simulink model "Xcvr_SSB_AM_2p5"  (Simulink 8.0)
settings: Solver=VariableStepDiscrete  SolverMode=SingleTasking  StartTime=0.0  StopTime=10  RelTol=1e-3
PreLoadFcn:
  | Fs=80e6;
  | 
  | phee=da_rom();
  | [phee_1,phee_2]=da_i2_rom();
  | 
  | Dcic=64;       % CIC decimation
  | Dfac=128;    % following DA filter decimation
  | N = 6;           %       (2^(N+1))=Dfac
  | Daudio=Dcic*Dfac;
  | Faudio=Fs/Daudio;
  | 
  | load info_filt_ssb_4
  | load Serial_Intfc_Stream_5
  | 
  | % AGC related
  | x=0.5:1/256:(1-1/256);
  | addr=(x-0.5)*256;
  | y=1./x;
values from neighbouring files (symbols this model uses):
  Serial_Interface = [0 0 0 0 0 0 0 0 0 0 0 0 ... (11390 elements, 2x5695)]    [Serial_Intfc_Stream_5.mat]
undefined symbols (not defined in the file or in its folder): get, sided, Two, xlipgetpartsetting
undefined symbols (not defined in the file): ssb_coef
libraries: xbsIndex_r4 x1305, dspsrcs4 x5, simulink x2, dspsigops x2, dspsnks4 x1
(part 3 of 11)

== system Xcvr_SSB_AM_2p5/Audio_and_Mode_Control/T_R_Delay ==
  note: ^ Inserted serial delay here
      | to delay Tx (to help preserve
      | length of iniial CW character, which
      | normally is clipped by about 13 ms).
  Tx_Rx_bit : Inport
  Delay : Inport  Port=2
  Constant1 : xbsIndex_r4/Constant  const=40  gui_display_data_type=Fixed-point  arith_type=Unsigned  n_bits=6  bin_pt=0  preci_type=Single  exp_width=8  frac_width=24  explicit_period=off  period=1  equ=P=C  opselect=C  inp2=PCIN>>17  opr=+  inp1=P  carry=CIN  dbl_ovrd=off  block_type=constant
      settings: block_version=12.1
  Constant2 : xbsIndex_r4/Constant  const=0  gui_display_data_type=Fixed-point  arith_type=Unsigned  n_bits=13  bin_pt=0  preci_type=Single  exp_width=8  frac_width=24  explicit_period=off  period=1  equ=P=C  opselect=C  inp2=PCIN>>17  opr=+  inp1=P  carry=CIN  dbl_ovrd=off  block_type=constant
      settings: block_version=12.1
  Counter : xbsIndex_r4/Counter  cnt_type=Free Running  cnt_to=0  operation=Down  start_count=0  cnt_by_val=1  arith_type=Unsigned  n_bits=12  bin_pt=0  load_pin=on  rst=off  en=on  explicit_period=off  period=1/Faudio  dbl_ovrd=off  use_behavioral_HDL=off  implementation=Fabric  block_type=counter
      settings: block_version=12.1
  Counter1 : xbsIndex_r4/Counter  cnt_type=Free Running  cnt_to=47  operation=Up  start_count=0  cnt_by_val=1  arith_type=Unsigned  n_bits=6  bin_pt=0  load_pin=off  rst=on  en=on  explicit_period=off  period=1  dbl_ovrd=off  use_behavioral_HDL=off  implementation=Fabric  block_type=counter
      settings: block_version=12.1
  Delay1 : xbsIndex_r4/Delay  rst=off  infoeditControl=Selection of Reset will increase slice count due to use of real FFs and instead of SRLs  en=off  latency=160  dbl_ovrd=off  reg_retiming=off  block_type=delay
      settings: block_version=9.2.00
  Delay2 : xbsIndex_r4/Delay  rst=off  infoeditControl=Selection of Reset will increase slice count due to use of real FFs and instead of SRLs  en=off  latency=1  dbl_ovrd=off  reg_retiming=off  block_type=delay
      settings: block_version=9.2.00
  Delay5 : xbsIndex_r4/Delay  rst=off  infoeditControl=Selection of Reset will increase slice count due to use of real FFs and instead of SRLs  en=off  latency=1  dbl_ovrd=off  reg_retiming=off  block_type=delay
      settings: block_version=9.2.00
  Inverter{1..4} (4 alike) : xbsIndex_r4/Inverter  en=off  latency=0  dbl_ovrd=off  block_type=inv
      settings: block_version=9.2.00
  Logical1 : xbsIndex_r4/Logical  logical_function=AND  inputs=2  en=off  latency=0  precision=Full  arith_type=Unsigned  n_bits=16  bin_pt=0  align_bp=on  dbl_ovrd=off  block_type=logical
      settings: block_version=12.1
  Logical2 : xbsIndex_r4/Logical  logical_function=AND  inputs=2  en=off  latency=0  precision=Full  arith_type=Unsigned  n_bits=16  bin_pt=0  align_bp=on  dbl_ovrd=off  block_type=logical
      settings: block_version=12.1
  Logical3 : xbsIndex_r4/Logical  logical_function=OR  inputs=2  en=off  latency=0  precision=Full  arith_type=Unsigned  n_bits=16  bin_pt=0  align_bp=on  dbl_ovrd=off  block_type=logical
      settings: block_version=12.1
  Logical4 : xbsIndex_r4/Logical  logical_function=OR  inputs=3  en=off  latency=0  precision=Full  arith_type=Unsigned  n_bits=16  bin_pt=0  align_bp=on  dbl_ovrd=off  block_type=logical
      settings: block_version=12.1
  Relational : xbsIndex_r4/Relational  mode=a=b  en=off  latency=0  dbl_ovrd=off  block_type=relational
      settings: block_version=9.2.00
  Relational1 : xbsIndex_r4/Relational  mode=a=b  en=off  latency=0  dbl_ovrd=off  block_type=relational
      settings: block_version=9.2.00
  Tx_Rx_D40 : Outport
  Tx_RX : Outport  Port=2
  Tx_RX_Delayed : Outport  Port=3
  wires:
  Tx_Rx_bit/1 -> Delay2/1, Inverter2/1, Logical4/1
  Delay2/1 -> Logical2/2, Logical4/2, Delay1/1
  Constant2/1 -> Relational/2
  Counter/1 -> Relational/1
  Relational/1 -> Inverter1/1
  Inverter1/1 -> Logical3/2, Logical4/3
  Logical3/1 -> Counter/3
  Delay/1 -> Counter/2
  Inverter2/1 -> Logical2/1
  Logical2/1 -> Counter/1, Logical3/1
  Logical4/1 -> Delay5/1
  Delay5/1 -> Tx_RX_Delayed/1, Logical1/1, Inverter3/1
  Counter1/1 -> Relational1/1
  Relational1/1 -> Logical1/2, Inverter4/1
  Inverter3/1 -> Counter1/1
  Constant1/1 -> Relational1/2
  Inverter4/1 -> Counter1/2
  Logical1/1 -> Tx_Rx_D40/1
  Delay1/1 -> Tx_RX/1

== system Xcvr_SSB_AM_2p5/RX Filters D=8192/CIC D64 ==
  note: Select Bits to feed subsequent filters
      | X1  46,44
      | X2  46,43
      | X4 46,42
      | X8 46,41
  I_in : Inport
  Q_in : Inport  Port=2
  CIC Filter : Subsystem  mask(CIC Filter){input_bitwidth=16, input_binpt=15, filter_type=Decimator, rate_change=64, stages=5, m=1, pipeline=on}
      mask prompts: input_bitwidth "Input Bit Width"; input_binpt "Input Binary Point"; filter_type "Filter Type"; rate_change "Sample Rate Change"; stages "Number of Stages"; m "Differential Delay"; pipeline "Pipeline Differentiators"
      mask help: Cascaded Integrated Comb (CIC) Filter
      mask init:
      | % CIC Single Channel v1.0
      | % Set Block Logo
      | sav_gcb=gcb;
      | [bg,fg] = xlcmap('XBlock',0);
      | iPos = get_param(sav_gcb,'Position');
      | iWidth=iPos(3)-iPos(1); iHeight=iPos(4)-iPos(2);
      | iCx=iWidth/2;
      | iCy=iHeight/2;
      | [logoX, logoY] = xlogo(iPos);
      | 
      | % Determine previous filter type and number of stages
      | prev_stages_list = find_system(sav_gcb, 'lookUnderMasks', 'all', 'FollowLinks', 'on', 'Regexp', 'on', 'Name', '^Integrator*'); %this is a cell array
      | prev_stages = length(prev_stages_list);
      | 
      | prev_filter_list = find_system(sav_gcb, 'lookUnderMasks', 'all', 'FollowLinks', 'on', 'Regexp', 'on', 'Name', '^Up Sample*'); %this is a cell array
      | if (isempty(prev_filter_list))
      |     prev_filter_list = find_system(sav_gcb, 'lookUnderMasks', 'all', 'FollowLinks', 'on', 'Regexp', 'on', 'Name', '^Down Sample*'); %this is a cell array
      |     if (isempty(prev_filter_list))
      |         errordlg('Previous Filter Type could not be determined')
      |     else
      |         prev_filter_type = 2;
      |     end
      | else
      |     prev_filter_type = 1;
      | end
      |   
      |   
      | % Print label on the block
      | if(filter_type == 2)
      |    cic_str = sprintf('%d-Stage\n CIC\n%d:1 Decimator',stages, rate_change);
      | else
      |    cic_str = sprintf('%d-Stage\n CIC\n1:%d Interpolator',stages, rate_change);	
      | end
      | 
      | % Make sure the entered values for stages and channels are positive integers
      | nstages = round(sum(abs(stages)));
      | 
      | % issue an error if the number of stages entered is zero
      | if (nstages == 0)
      | 	nstages = prev_stages;
      | 	errordlg('Number of Stages must be more than zero')
      | end
      | 
      | if (nstages == prev_stages) & (filter_type == prev_filter_type)
      |     return
      | end
      | 
      | if(filter_type == 2) % Decimator
      |    if (prev_filter_type == 1) % was interpolator so turn to decimator
      |        for i= 2:prev_stages,
      | 	      delete_line(sav_gcb, ['Integrator' int2str(i-1) '/' int2str(1)], ['Integrator' int2str(i) '/' int2str(1)]);
      | 	      delete_line(sav_gcb, ['Differentiator' int2str(i-1) '/' int2str(1)], ['Differentiator' int2str(i) '/' int2str(1)]);
      |        end
      | 
      |        % disconnect the last blocks in the two sections
      |        delete_line(sav_gcb, ['Differentiator' int2str(prev_stages) '/' int2str(1)], ['Up Sample/1']);
      |        delete_line(sav_gcb, ['Integrator' int2str(prev_stages) '/' int2str(1)], 'Out1/1');
      | 	
      | 	   % delete the line from the Up sampler to the Integrator
      | 	   delete_line(sav_gcb, 'Up Sample/1', 'Integrator1/1'); 
      | 	   delete_line(sav_gcb, 'In1/1', 'Differentiator1/1'); 
      | 	   
      | 	   % Delete the Up Sampler and then replace with an Down Sampler
      | 	   pup = get_param([sav_gcb '/Up Sample'], 'position');
      | 	   delete_block([sav_gcb '/Up Sample']);
      | 	   load_system('xbsIndex_r4');
      | 	   add_block('xbsIndex_r4/Down Sample', [sav_gcb '/Down Sample'], 'sample_ratio', 'rate_change','sample_phase', 'First Value of Frame', 'position', [pup(1), pup(2), pup(3),pup(4)]);
      | 	   
      | 	   % Switch the Integrators and Decimators around
      | 	   for i=1:prev_stages,
      | 		   tempi = get_param([sav_gcb '/Integrator' int2str(i)], 'position');
      | 	       tempd = get_param([sav_gcb '/Differentiator' int2str(i)], 'position');
      | 		   set_param([sav_gcb '/Differentiator' int2str(i)], 'position', [tempi(1), tempi(2), tempi(3), tempi(4)], 'output_bitwidth', 'ceil(stages*log2(rate_change*m) + input_bitwidth)');
      | 		   set_param([sav_gcb '/Integrator' int2str(i)], 'position', [tempd(1), tempd(2), tempd(3), tempd(4)]);
      | 	   end
      | 	   	   	
      | 	   % add back in the lines
      |        add_line(sav_gcb, 'In1/1', 'Integrator1/1', 'autorouting', 'on');
      | 	   add_line(sav_gcb, ['Integrator' int2str(prev_stages) '/1'], 'Down Sample/1', 'autorouting', 'on');
      | 	   add_line(sav_gcb, 'Down Sample/1', 'Differentiator1/1', 'autorouting', 'on');
      | 	   add_line(sav_gcb, ['Differentiator' int2str(prev_stages) '/1'], 'Out1/1', 'autorouting', 'on');
      | 	   for i= 2:prev_stages,
      |           add_line(sav_gcb, ['Integrator' int2str(i-1) '/1'], ['Integrator' int2str(i) '/' int2str(1)], 'autorouting', 'on');
      |           add_line(sav_gcb, ['Differentiator' int2str(i-1) '/1'], ['Differentiator' int2str(i) '/' int2str(1)], 'autorouting', 'on');
      | 	   end
      | 		
      |        %Set the Output bit widths of Differentiator and Integrator stages
      |        set_param([sav_gcb '/Differentiator1'], 'output_bitwidth', 'ceil(stages*log2(rate_change*m) + input_bitwidth)');
      | 	   	   %Set the Output bit width of Integrator stages
      | 	   %Calculate the Interpolator Integrator Output Bit Growth
      |        for i= 1:prev_stages,
      | 			 j = nstages+i;
      | 	         set_param([sav_gcb '/Integrator' int2str(i)], 'output_bitwidth', 'ceil(stages*log2(rate_change*m) + input_bitwidth)');
      |              set_param([sav_gcb '/Differentiator' int2str(i)], 'output_bitwidth', 'ceil(stages*log2(rate_change*m) + input_bitwidth)');
      | 	   end
      | 	   
      |    end
      |    
      |    if (nstages ~= prev_stages)
      |     
      |        % disconnect all the wires from all the blocks
      |        for i= 2:prev_stages,
      | 	      delete_line(sav_gcb, ['Integrator' int2str(i-1) '/' int2str(1)], ['Integrator' int2str(i) '/' int2str(1)]);
      | 	      delete_line(sav_gcb, ['Differentiator' int2str(i-1) '/' int2str(1)], ['Differentiator' int2str(i) '/' int2str(1)]);
      |        end
      | 
      |        % disconnect the last blocks in the two sections
      |        delete_line(sav_gcb, ['Integrator' int2str(prev_stages) '/' int2str(1)], ['Down Sample/1']);
      |        delete_line(sav_gcb, ['Differentiator' int2str(prev_stages) '/' int2str(1)], 'Out1/1');
      | 	
      | 	   % delete the line from the down sampler to the differentiator
      | 	   delete_line(sav_gcb, 'Down Sample/1', 'Differentiator1/1');
      | 	
      | 	   % Remove all the blocks except the first one (as we always will have one)
      |        for i=2:prev_stages,
      | 		  delete_block([sav_gcb '/Differentiator' int2str(i)]);
      | 	      delete_block([sav_gcb '/Integrator' int2str(i)]);
      |        end
      | 	   
      | 	   %Set the Output bit width of Differentiator stages
      |        set_param([sav_gcb '/Differentiator1'], 'output_bitwidth', 'ceil(stages*log2(rate_change*m) + input_bitwidth)');
      | 	   
      | 	   % collect data on the position of existing blocks
      | 	   pi = get_param([sav_gcb '/Integrator1'], 'position');
      | 	   pd = get_param([sav_gcb '/Differentiator1'], 'position');
      | 	   set_param([sav_gcb '/Differentiator1'], 'position', [pi(1)+(nstages+1)*80, pd(2), pi(3)+(nstages+1)*80, pd(4)]);
      | 	   pd = get_param([sav_gcb '/Differentiator1'], 'position');
      | 	
      | 	   % move the current blocks to accomadate for new blocks to be added 
      | 	   pds = get_param([sav_gcb '/Down Sample'], 'position');
      | 	   set_param([sav_gcb '/Down Sample'], 'position', [pi(1)+(nstages)*80, pds(2), pi(3)+(nstages)*80, pds(4)]);
      | 	   
      | 	   po = get_param([sav_gcb '/Out1'], 'position');
      | 	   set_param([sav_gcb '/Out1'], 'position', [pd(1)+(nstages+1)*80, po(2), pd(1)+(po(3)-po(1))+(nstages+1)*80, po(4)]);	
      | 	
      | 	   % add back in the line between the Down Sampler and the 1st Differentiator
      |        add_line(sav_gcb, 'Down Sample/1', ['Differentiator1/' int2str(1)], 'autorouting', 'on');
      | 
      | 	   % Only add blocks if more than one stage is required
      | 	   if (nstages ~= 1)
      | 		
      | 	       % Add in a copy of the first block to make up the required number of stages
      |            for i=2:nstages,
      |                add_block([sav_gcb '/Integrator1'], [sav_gcb '/Integrator' int2str(i)], 'position', [pi(1)+(i-1)*80, pi(2), pi(3)+(i-1)*80, pi(4)]);
      | 		       add_block([sav_gcb '/Differentiator1'], [sav_gcb '/Differentiator' int2str(i)], 'position', [pd(1)+(i-1)*80, pd(2), pd(3)+(i-1)*80, pd(4)]);
      | 	       end
      | 		
      | 	       % Connect up the wires to each block use autorouting
      |            for i= 2:nstages,
      |  		       add_line(sav_gcb, ['Integrator' int2str(i-1) '/' int2str(1)], ['Integrator' int2str(i) '/' int2str(1)], 'autorouting', 'on');
      | 	           add_line(sav_gcb, ['Differentiator' int2str(i-1) '/' int2str(1)], ['Differentiator' int2str(i) '/' int2str(1)], 'autorouting', 'on');
      |            end
      | 	    end
      | 	       % Connect the last blocks in the two sections
      |            add_line(sav_gcb, ['Integrator' int2str(nstages) '/' int2str(1)], ['Down Sample/1'], 'autorouting', 'on');
      |            add_line(sav_gcb, ['Differentiator' int2str(nstages) '/' int2str(1)], ['Out1/1'], 'autorouting', 'on');
      |    end
      | 
      | else % Interpolator
      |    
      | 	
      | 	if (prev_filter_type == 2) % was decimator so turn to interpolator
      | 	
      | 	  % disconnect all the wires from all the blocks
      |        for i= 2:prev_stages,
      | 	      delete_line(sav_gcb, ['Integrator' int2str(i-1) '/' int2str(1)], ['Integrator' int2str(i) '/' int2str(1)]);
      | 	      delete_line(sav_gcb, ['Differentiator' int2str(i-1) '/' int2str(1)], ['Differentiator' int2str(i) '/' int2str(1)]);
      |        end
      | 
      |        % disconnect the last blocks in the two sections
      |        delete_line(sav_gcb, ['Integrator' int2str(prev_stages) '/' int2str(1)], ['Down Sample/1']);
      |        delete_line(sav_gcb, ['Differentiator' int2str(prev_stages) '/' int2str(1)], 'Out1/1');
      | 	
      | 	   % delete the line from the down sampler to the Differentiator
      | 	   delete_line(sav_gcb, 'Down Sample/1', 'Differentiator1/1'); 
      | 	   delete_line(sav_gcb, 'In1/1', 'Integrator1/1'); 
      | 	   
      | 	   % Delete the Down Sampler and then replace with a Up Sampler
      | 	   pdwn = get_param([sav_gcb '/Down Sample'], 'position');
      | 	   delete_block([sav_gcb '/Down Sample']);
      | 	   load_system('xbsIndex_r4');
      | 	   add_block('xbsIndex_r4/Up Sample', [sav_gcb '/Up Sample'], 'sample_ratio', 'rate_change', 'position', [pdwn(1), pdwn(2), pdwn(3), pdwn(4)]);
      | 	   
      | 	   % Switch the Integrators and Decimators around
      | 	   for i=1:prev_stages,
      | 		   tempi = get_param([sav_gcb '/Integrator' int2str(i)], 'position');
      | 	       tempd = get_param([sav_gcb '/Differentiator' int2str(i)], 'position');
      | 		   set_param([sav_gcb '/Differentiator' int2str(i)], 'position', [tempi(1), tempi(2), tempi(3), tempi(4)], 'output_bitwidth', [int2str(i) '+ input_bitwidth']);
      | 		   set_param([sav_gcb '/Integrator' int2str(i)], 'position', [tempd(1), tempd(2), tempd(3), tempd(4)]);
      | 	   end
      | 	   	   	
      | 	   % add back in the lines
      |        add_line(sav_gcb, 'In1/1', 'Differentiator1/1', 'autorouting', 'on');
      | 	   add_line(sav_gcb, ['Differentiator' int2str(prev_stages) '/1'], 'Up Sample/1', 'autorouting', 'on');
      | 	   add_line(sav_gcb, 'Up Sample/1', 'Integrator1/1', 'autorouting', 'on');
      | 	   add_line(sav_gcb, ['Integrator' int2str(prev_stages) '/1'], 'Out1/1', 'autorouting', 'on');
      | 	   for i= 2:prev_stages,
      |           add_line(sav_gcb, ['Integrator' int2str(i-1) '/1'], ['Integrator' int2str(i) '/1'], 'autorouting', 'on');
      |           add_line(sav_gcb, ['Differentiator' int2str(i-1) '/1'], ['Differentiator' int2str(i) '/1'], 'autorouting', 'on');
      | 	   end
      | 	   
      | 	   %Set the Output bit width of Integrator stages
      | 	   %Calculate the Interpolator Integrator Output Bit Growth
      |        for i= 1:prev_stages,
      | 			 j = nstages+i;
      | 	         set_param([sav_gcb '/Integrator' int2str(i)], 'output_bitwidth', ['ceil(log2(2^(2*stages-' int2str(j) ')*(rate_change*m)^(' int2str(j) '-stages)) + input_bitwidth)']);
      | 	   end
      | 		
      |    end
      |    
      | 	
      | 	if (nstages ~= prev_stages)
      |     
      |        % disconnect all the wires from all the blocks
      |        for i= 2:prev_stages,
      | 	      delete_line(sav_gcb, ['Integrator' int2str(i-1) '/' int2str(1)], ['Integrator' int2str(i) '/' int2str(1)]);
      | 	      delete_line(sav_gcb, ['Differentiator' int2str(i-1) '/' int2str(1)], ['Differentiator' int2str(i) '/' int2str(1)]);
      |        end
      | 
      |        % disconnect the last blocks in the two sections
      |        delete_line(sav_gcb, ['Differentiator' int2str(prev_stages) '/' int2str(1)], ['Up Sample/1']);
      |        delete_line(sav_gcb, ['Integrator' int2str(prev_stages) '/' int2str(1)], 'Out1/1');
      |        
      | 	
      | 	   % delete the line from the Up sampler to the Integrator1 for movement later
      | 	   delete_line(sav_gcb, 'Up Sample/1', 'Integrator1/1'); 
      | 	
      | 	   % Remove all the blocks except the first one (as we always will have one)
      |        for i=2:prev_stages,
      | 		  delete_block([sav_gcb '/Differentiator' int2str(i)]);
      | 	      delete_block([sav_gcb '/Integrator' int2str(i)]);
      |        end
      | 	
      | 	   %Set the Output bit width of first Differentiator stage (other are set as copies of this block)
      |        set_param([sav_gcb '/Differentiator1'], 'output_bitwidth', '1 + input_bitwidth');
      | 	   
      | 	   % collect data on the position of existing blocks
      | 	   pi = get_param([sav_gcb '/Integrator1'], 'position');
      | 	   pd = get_param([sav_gcb '/Differentiator1'], 'position');
      | 	   set_param([sav_gcb '/Integrator1'], 'position', [pd(1)+(nstages+1)*80, pi(2), pd(3)+(nstages+1)*80, pi(4)]);
      | 	   pi = get_param([sav_gcb '/Integrator1'], 'position');
      | 	
      | 	   % move the current blocks to accomadate for new blocks to be added 
      | 	   pus = get_param([sav_gcb '/Up Sample'], 'position');
      | 	   set_param([sav_gcb '/Up Sample'], 'position', [pd(1)+(nstages)*80, pus(2), pd(3)+(nstages)*80, pus(4)]);
      | 	
      | 	   po = get_param([sav_gcb '/Out1'], 'position');
      |        set_param([sav_gcb '/Out1'], 'position', [pi(1)+(nstages+1)*80, po(2), pi(1)+(po(3)-po(1))+(nstages+1)*80, po(4)]);	
      |       
      | 	
      | 	   % add back in the line between the Up Sampler and the 1st Integrator1
      | 	   add_line(sav_gcb, 'Up Sample/1', 'Integrator1/1', 'autorouting', 'on');
      | 	   
      | 	   % Only add blocks if more than one stage is required
      | 	   if (nstages ~= 1)
      | 		
      | 	       % Add in a copy of the first block to make up the required number of stages
      |            for i=2:nstages,
      |                add_block([sav_gcb '/Integrator1'], [sav_gcb '/Integrator' int2str(i)], 'position', [pi(1)+(i-1)*80, pi(2), pi(3)+(i-1)*80, pi(4)]);
      | 		       add_block([sav_gcb '/Differentiator1'], [sav_gcb '/Differentiator' int2str(i)], 'position', [pd(1)+(i-1)*80, pd(2), pd(3)+(i-1)*80, pd(4)], 'output_bitwidth', [int2str(i) '+ input_bitwidth']);
      | 	       end
      | 		
      | 	       % Connect up the wires to each block use autorouting
      |            for i= 2:nstages,
      |  		       add_line(sav_gcb, ['Integrator' int2str(i-1) '/' int2str(1)], ['Integrator' int2str(i) '/' int2str(1)], 'autorouting', 'on');
      | 	           add_line(sav_gcb, ['Differentiator' int2str(i-1) '/' int2str(1)], ['Differentiator' int2str(i) '/' int2str(1)], 'autorouting', 'on');
      |            end
      | 	    end
      | 	       % Connect the last blocks in the two sections
      |            add_line(sav_gcb, ['Differentiator' int2str(nstages) '/1'], ['Up Sample/1'], 'autorouting', 'on');
      |            add_line(sav_gcb, ['Integrator' int2str(nstages) '/1'], ['Out1/1'], 'autorouting', 'on');
      | 		   
      | 	     %Set the Output bit width of Integrator stages
      | 	     %Calculate the Interpolator Integrator Output Bit Growth
      |           for i= 1:nstages,
      | 			 j = nstages+i;
      | 	         set_param([sav_gcb '/Integrator' int2str(i)], 'output_bitwidth', ['ceil(log2(2^(2*stages-' int2str(j) ')*(rate_change*m)^(' int2str(j) '-stages)) + input_bitwidth)']);
      | 	      end
      |    end
      | 	  
      | end
      | 
      | 
      | % Set the pipelining to ON or OFF on the differentiators
      | if (pipeline == 0)
      | 	for i= 1:nstages
      | 		set_param([sav_gcb '/Differentiator' int2str(i), '/AddSub'], 'latency', '0')
      | 	end
      | else
      | 	for i= 1:nstages
      | 		set_param([sav_gcb '/Differentiator' int2str(i), '/AddSub'], 'latency' ,'1')
      | 	end
      | end
      settings: CopyFcn=set_param(gcb, 'MaskSelfModifiable', 'on', 'LinkStatus', 'none');
      mask Help: eval('');xlDoc('-book','sysgen','-topic','CIC_Filter');
      mask TypeOptions filter_type: Interpolator | Decimator
      mask TypeOptions m: 1 | 2 | 3 | 4
      mask Display:
      | patch([0 iWidth iWidth 0],[0 0 iHeight iHeight] , bg);
      | patch(logoX,logoY , fg);
      | plot([0 0 iWidth iWidth 0], [0 iHeight iHeight 0 0]);
      | disp(cic_str)
  CIC Filter1 : Subsystem  mask(CIC Filter){input_bitwidth=16, input_binpt=15, filter_type=Decimator, rate_change=64, stages=5, m=1, pipeline=on}
      mask prompts: input_bitwidth "Input Bit Width"; input_binpt "Input Binary Point"; filter_type "Filter Type"; rate_change "Sample Rate Change"; stages "Number of Stages"; m "Differential Delay"; pipeline "Pipeline Differentiators"
      mask help: Cascaded Integrated Comb (CIC) Filter
      mask init: same as Xcvr_SSB_AM_2p5/RX Filters D=8192/CIC D64/CIC Filter
      settings: CopyFcn=set_param(gcb, 'MaskSelfModifiable', 'on', 'LinkStatus', 'none');
      mask Help: eval('');xlDoc('-book','sysgen','-topic','CIC_Filter');
      mask TypeOptions filter_type: Interpolator | Decimator
      mask TypeOptions m: 1 | 2 | 3 | 4
      mask Display:
      | patch([0 iWidth iWidth 0],[0 0 iHeight iHeight] , bg);
      | patch(logoX,logoY , fg);
      | plot([0 0 iWidth iWidth 0], [0 iHeight iHeight 0 0]);
      | disp(cic_str)
  Convert1 : xbsIndex_r4/Convert  gui_display_data_type=Fixed-point  arith_type="Signed  (2's comp)"  n_bits=21  bin_pt=20  float_type=Single  exp_bits=8  fraction_bits=24  quantization="Round  (unbiased: +/- Inf)"  overflow=Saturate  en=off  latency=1  dbl_ovrd=off  pipeline=off  block_type=convert
      settings: block_version=9.2.00
  Convert2 : xbsIndex_r4/Convert  gui_display_data_type=Fixed-point  arith_type="Signed  (2's comp)"  n_bits=21  bin_pt=20  float_type=Single  exp_bits=8  fraction_bits=24  quantization="Round  (unbiased: +/- Inf)"  overflow=Saturate  en=off  latency=1  dbl_ovrd=off  pipeline=off  block_type=convert
      settings: block_version=9.2.00
  OverLoad_Det : Subsystem
  Reinterpret  X1a : xbsIndex_r4/Reinterpret  force_arith_type=on  arith_type="Signed  (2's comp)"  force_bin_pt=on  bin_pt=44  block_type=reinterpret
      settings: infoedit="Changes signal type without altering the binary representation.   You can changed the signal between signed and unsigned, and relocate the binary point.<br><br>Hardware notes: In hardware this block costs nothing.<br><br>Example:  Suppose the input is 6 bits wide, signed, with 2 fractional bits, and the output is forced to unsigned with 0 fractional bits.  Then an input of -2.0 (1110.00 in binary 2's complement) becomes an output of 56 (111000 in binary)."  block_version=9.2.00
  Reinterpret1 : xbsIndex_r4/Reinterpret  force_arith_type=on  arith_type="Signed  (2's comp)"  force_bin_pt=on  bin_pt=44  block_type=reinterpret
      settings: infoedit="Changes signal type without altering the binary representation.   You can changed the signal between signed and unsigned, and relocate the binary point.<br><br>Hardware notes: In hardware this block costs nothing.<br><br>Example:  Suppose the input is 6 bits wide, signed, with 2 fractional bits, and the output is forced to unsigned with 0 fractional bits.  Then an input of -2.0 (1110.00 in binary 2's complement) becomes an output of 56 (111000 in binary)."  block_version=9.2.00
  I_Out : Outport
  Q_Out : Outport  Port=2
  CIC_Ovl : Outport  Port=3
  wires:
  CIC Filter/1(Out1) -> Reinterpret  X1a/1
  Reinterpret  X1a/1 -> Convert2/1
  I_in/1 -> CIC Filter/1(In1)
  Q_in/1 -> CIC Filter1/1(In1)
  Convert2/1 -> I_Out/1, OverLoad_Det/1(In1)  "I_X1"
  CIC Filter1/1(Out1) -> Reinterpret1/1
  Reinterpret1/1 -> Convert1/1
  OverLoad_Det/1(Out1) -> CIC_Ovl/1
  Convert1/1 -> Q_Out/1  "Q_X1"

== system Xcvr_SSB_AM_2p5/RX Filters D=8192/DA_Ovl_Det ==
  In1 : Inport
  Constant : xbsIndex_r4/Constant  const=0  gui_display_data_type=Fixed-point  arith_type=Unsigned  n_bits=8  bin_pt=0  preci_type=Single  exp_width=8  frac_width=24  explicit_period=off  period=1  equ=P=C  opselect=C  inp2=PCIN>>17  opr=+  inp1=P  carry=CIN  dbl_ovrd=off  block_type=constant
      settings: block_version=9.2.00
  Counter : xbsIndex_r4/Counter  cnt_type=Free Running  cnt_to=Inf  operation=Up  start_count=0  cnt_by_val=1  arith_type=Unsigned  n_bits=8  bin_pt=0  load_pin=off  rst=off  en=off  explicit_period=on  period=8192/Fs  dbl_ovrd=off  use_behavioral_HDL=off  implementation=Fabric  use_rpm=off  block_type=counter
      settings: block_version=9.2.00
  Inverter{,1..3} (4 alike) : xbsIndex_r4/Inverter  en=off  latency=0  dbl_ovrd=off  block_type=inv
      settings: block_version=9.2.00
  Logical : xbsIndex_r4/Logical  logical_function=AND  inputs=4  en=off  latency=0  precision=Full  arith_type=Unsigned  n_bits=16  bin_pt=0  align_bp=on  dbl_ovrd=off  block_type=logical
      settings: block_version=9.2.00
  Logical1 : xbsIndex_r4/Logical  logical_function=AND  inputs=4  en=off  latency=0  precision=Full  arith_type=Unsigned  n_bits=16  bin_pt=0  align_bp=on  dbl_ovrd=off  block_type=logical
      settings: block_version=9.2.00
  Logical2 : xbsIndex_r4/Logical  logical_function=OR  inputs=2  en=off  latency=1  precision=Full  arith_type=Unsigned  n_bits=16  bin_pt=0  align_bp=on  dbl_ovrd=off  block_type=logical
      settings: block_version=9.2.00
  Logical3 : xbsIndex_r4/Logical  logical_function=OR  inputs=2  en=off  latency=0  precision=Full  arith_type=Unsigned  n_bits=16  bin_pt=0  align_bp=on  dbl_ovrd=off  block_type=logical
      settings: block_version=9.2.00
  Register : xbsIndex_r4/Register  init=0  rst=on  en=off  dbl_ovrd=off  block_type=register
      settings: block_version=9.2.00
  Relational : xbsIndex_r4/Relational  mode=a=b  en=off  latency=0  dbl_ovrd=off  block_type=relational
      settings: block_version=9.2.00
  Slice : xbsIndex_r4/Slice  nbits=1  boolean_output=on  mode=Upper Bit Location + Width  bit1=0  base1=MSB of Input  bit0=0  base0=LSB of Input  dbl_ovrd=off  block_type=slice
      settings: infoedit="Extracts a given range of bits from each input sample and presents it at the output.  The output type is ordinarily unsigned with binary point at zero, but can be Boolean when the slice is one bit wide.<P><P>Hardware notes: In hardware this block costs nothing."  block_version=9.2.00
  Slice1 : xbsIndex_r4/Slice  nbits=1  boolean_output=on  mode=Upper Bit Location + Width  bit1=-1  base1=MSB of Input  bit0=0  base0=LSB of Input  dbl_ovrd=off  block_type=slice
      settings: infoedit="Extracts a given range of bits from each input sample and presents it at the output.  The output type is ordinarily unsigned with binary point at zero, but can be Boolean when the slice is one bit wide.<P><P>Hardware notes: In hardware this block costs nothing."  block_version=9.2.00
  Slice2 : xbsIndex_r4/Slice  nbits=1  boolean_output=on  mode=Upper Bit Location + Width  bit1=-2  base1=MSB of Input  bit0=0  base0=LSB of Input  dbl_ovrd=off  block_type=slice
      settings: infoedit="Extracts a given range of bits from each input sample and presents it at the output.  The output type is ordinarily unsigned with binary point at zero, but can be Boolean when the slice is one bit wide.<P><P>Hardware notes: In hardware this block costs nothing."  block_version=9.2.00
  Slice3 : xbsIndex_r4/Slice  nbits=1  boolean_output=on  mode=Upper Bit Location + Width  bit1=-3  base1=MSB of Input  bit0=0  base0=LSB of Input  dbl_ovrd=off  block_type=slice
      settings: infoedit="Extracts a given range of bits from each input sample and presents it at the output.  The output type is ordinarily unsigned with binary point at zero, but can be Boolean when the slice is one bit wide.<P><P>Hardware notes: In hardware this block costs nothing."  block_version=9.2.00
  Out1 : Outport
  wires:
  Slice/1 -> Inverter/1, Logical1/1
  In1/1 -> Slice/1, Slice1/1, Slice2/1, Slice3/1
  Inverter/1 -> Logical/1
  Slice1/1 -> Logical/2, Inverter1/1
  Slice2/1 -> Logical/3, Inverter2/1
  Slice3/1 -> Logical/4, Inverter3/1
  Inverter1/1 -> Logical1/2
  Inverter2/1 -> Logical1/3
  Inverter3/1 -> Logical1/4
  Logical1/1 -> Logical2/2
  Logical/1 -> Logical2/1
  Logical2/1 -> Logical3/1
  Logical3/1 -> Register/1
  Register/1 -> Out1/1, Logical3/2
  Relational/1 -> Register/2
  Counter/1 -> Relational/1
  Constant/1 -> Relational/2

== system Xcvr_SSB_AM_2p5/RX Filters D=8192/Decimating Filter DC Optimized in Accumulator Plus Pipelined Stage Control. Improved dynamic  range.  ==
  Real_In : Inport
  Imag_In : Inport  Port=2
  Dfac : Inport  Port=3
  D=2 Bit Serial Filter Core with Piplined RAM Based SR : Subsystem
  Interstage  Interface1 : Subsystem
  Real_Imag_Demux1 : Subsystem
  Reinterpret2 : xbsIndex_r4/Reinterpret  force_arith_type=on  arith_type="Signed  (2's comp)"  force_bin_pt=on  bin_pt=20  block_type=reinterpret
      settings: infoedit="Changes signal type without altering the binary representation.   You can changed the signal between signed and unsigned, and relocate the binary point.<br><br>Hardware notes: In hardware this block costs nothing.<br><br>Example:  Suppose the input is 6 bits wide, signed, with 2 fractional bits, and the output is forced to unsigned with 0 fractional bits.  Then an input of -2.0 (1110.00 in binary 2's complement) becomes an output of 56 (111000 in binary)."  block_version=9.2.00
  Reinterpret3 : xbsIndex_r4/Reinterpret  force_arith_type=on  arith_type="Signed  (2's comp)"  force_bin_pt=on  bin_pt=0  block_type=reinterpret
      settings: infoedit="Changes signal type without altering the binary representation.   You can changed the signal between signed and unsigned, and relocate the binary point.<P><P>Hardware notes: In hardware this block costs nothing.<P><P>Example:  Suppose the input is 6 bits wide, signed, with 2 fractional bits, and the output is forced to unsigned with 0 fractional bits.  Then an input of -2.0 (1110.00 in binary 2's complement) becomes an output of 56 (111000 in binary)."  block_version=9.2.00
  Reinterpret4 : xbsIndex_r4/Reinterpret  force_arith_type=on  arith_type="Signed  (2's comp)"  force_bin_pt=on  bin_pt=20  block_type=reinterpret
      settings: infoedit="Changes signal type without altering the binary representation.   You can changed the signal between signed and unsigned, and relocate the binary point.<br><br>Hardware notes: In hardware this block costs nothing.<br><br>Example:  Suppose the input is 6 bits wide, signed, with 2 fractional bits, and the output is forced to unsigned with 0 fractional bits.  Then an input of -2.0 (1110.00 in binary 2's complement) becomes an output of 56 (111000 in binary)."  block_version=9.2.00
  Reinterpret5 : xbsIndex_r4/Reinterpret  force_arith_type=on  arith_type="Signed  (2's comp)"  force_bin_pt=on  bin_pt=0  block_type=reinterpret
      settings: infoedit="Changes signal type without altering the binary representation.   You can changed the signal between signed and unsigned, and relocate the binary point.<P><P>Hardware notes: In hardware this block costs nothing.<P><P>Example:  Suppose the input is 6 bits wide, signed, with 2 fractional bits, and the output is forced to unsigned with 0 fractional bits.  Then an input of -2.0 (1110.00 in binary 2's complement) becomes an output of 56 (111000 in binary)."  block_version=9.2.00
  Relational : xbsIndex_r4/Relational  mode=a=b  en=off  latency=0  dbl_ovrd=off  block_type=relational
      settings: block_version=9.2.00
  Stage Control with Pipe : Subsystem
  Terminator1 : Terminator
  Real_Out : Outport
  Imag_Out : Outport  Port=2
  wires:
  Reinterpret4/1 -> Imag_Out/1
  Stage Control with Pipe/2(SR_addr) -> D=2 Bit Serial Filter Core with Piplined RAM Based SR/3(SR_addr)
  Stage Control with Pipe/3(Real_Imag) -> Interstage  Interface1/7(Real_Imag), Real_Imag_Demux1/3(Real_Imag)
  Stage Control with Pipe/1(AB_Addr) -> Interstage  Interface1/5(AB_Addr)
  Stage Control with Pipe/5(Write_OK) -> Interstage  Interface1/8(Write_OK)
  D=2 Bit Serial Filter Core with Piplined RAM Based SR/1(Yn) -> Real_Imag_Demux1/1(Yn), Interstage  Interface1/1(Previous Stage)
  D=2 Bit Serial Filter Core with Piplined RAM Based SR/2(Valid) -> Interstage  Interface1/2(Write), Real_Imag_Demux1/2(Valid_In)
  Stage Control with Pipe/6(Start) -> D=2 Bit Serial Filter Core with Piplined RAM Based SR/4(Start)
  Stage Control with Pipe/7(Stage) -> Relational/1
  Relational/1 -> Real_Imag_Demux1/4(Stage_Sel)
  Real_In/1 -> Reinterpret3/1
  Real_Imag_Demux1/1(Real) -> Reinterpret2/1  "Real"
  Real_Imag_Demux1/2(Imag) -> Reinterpret4/1
  Real_Imag_Demux1/3(Valid) -> Terminator1/1  "Valid"
  Reinterpret3/1 -> Interstage  Interface1/3(Real_In)
  Reinterpret5/1 -> Interstage  Interface1/4(Imag_In)
  Imag_In/1 -> Reinterpret5/1
  Stage Control with Pipe/4(Stage>0) -> Interstage  Interface1/6(Stage>0)
  Interstage  Interface1/1(Xn) -> D=2 Bit Serial Filter Core with Piplined RAM Based SR/1(Xn)
  Interstage  Interface1/2(Xn-1) -> D=2 Bit Serial Filter Core with Piplined RAM Based SR/2(Xn-1)
  Reinterpret2/1 -> Real_Out/1
  Dfac/1 -> Relational/2

== system Xcvr_SSB_AM_2p5/RX Filters D=8192/Fs_probe ==
  In1 : Inport
  Probe : Probe  ProbeWidth=off  ProbeComplexSignal=off
  Product : Product  Inputs=/  RndMeth=Zero
  Selector : Selector  InputPortWidth=2  IndexOptions=Index vector (dialog)  Indices=1  OutputSizes=1
  Out1 : Outport
  wires:
  Selector/1 -> Product/1
  Probe/1 -> Selector/1
  In1/1 -> Probe/1
  Product/1 -> Out1/1

== system Xcvr_SSB_AM_2p5/SSB / AM Mod_Demod WCS/128 Tap FIR with  Writable Coefficient Store ==
  note: [15 14 13 12 .... 3 2 1 0] [5 4 3 2 1 0] [Bank_Sel] [Reset], [WE] X
  note: 16 Data 6 Address Bank Select Reset Write Enable X
  note: 25 24 23 22 ....13 12 11 10 9 8 7 6 5 4 3 2 1 0
  note: Added delay 7/31/2016
  note: To load WCS:
      | 1) Set Reset Bit then in a loop...
      | 2) With both Reset and WE set,
      | load 6 address and 16 Data bits. 64X for entire RAM.
      | 3) Lower both Reset and WE.
      | Yes one bit could do the job.
  I_In : Inport
  Q_In : Inport  Port=2
  Data_26 : Inport  Port=3
  WR_COEF_RAM : Inport  Port=4
  Tx_Rx_Delayed : Inport  Port=5
  2 channel (IQ)  SHARED MPY MAC with Writable Coefficient Store : Subsystem  mask(2n-tap Linear Phase MAC FIR Filter){coef=ssb_coef, coef_n_bits=16, coef_bin_pt=16, smpl_n_bits=18, smpl_bin_pt=17, smpl_period=Daudio/Fs}
      mask prompts: coef "Coefficients_1"; coef_n_bits "Number of Bits per Coefficient"; coef_bin_pt "Binary Point for Coefficient"; smpl_n_bits "Number of Bits per Input Sample"; smpl_bin_pt "Binary Point for Input Samples"; smpl_period "Input Sample Period"
      mask help:
      | Linear phase MAC-based FIR filter with 2*n coefficients.
      | Design exploits even coefficient symmetry.
      mask init:
      | dstr = sprintf('%d tap',length(coef));
  Address_Slice : xbsIndex_r4/Slice  nbits=6  boolean_output=off  mode=Lower Bit Location + Width  bit1=-17  base1=LSB of Input  bit0=4  base0=LSB of Input  dbl_ovrd=off  block_type=slice
      settings: block_version=12.1
  Bank_Sel : xbsIndex_r4/Slice  nbits=1  boolean_output=on  mode=Lower Bit Location + Width  bit1=-17  base1=LSB of Input  bit0=3  base0=LSB of Input  dbl_ovrd=off  block_type=slice
      settings: block_version=12.1
  Data_Slice : xbsIndex_r4/Slice  nbits=16  boolean_output=off  mode=Lower Bit Location + Width  bit1=-17  base1=LSB of Input  bit0=10  base0=LSB of Input  dbl_ovrd=off  block_type=slice
      settings: block_version=12.1
  Down Sample : xbsIndex_r4/Down Sample  sample_ratio=1024/4  sample_phase="Last Value of Frame  (most efficient)"  en=off  latency=1  dbl_ovrd=off  block_type=dsamp
      settings: block_version=9.2.00
  Down Sample1 : xbsIndex_r4/Down Sample  sample_ratio=256  sample_phase=First Value of Frame  en=off  latency=0  dbl_ovrd=off  block_type=dsamp
      settings: block_version=9.2.00
  Information_Filter_Transient_Suppressor : Subsystem
  Logical : xbsIndex_r4/Logical  logical_function=OR  inputs=2  en=off  latency=0  precision=Full  arith_type=Unsigned  n_bits=16  bin_pt=0  align_bp=on  dbl_ovrd=off  block_type=logical
      settings: block_version=9.2.00
  Logical1 : xbsIndex_r4/Logical  logical_function=AND  inputs=2  en=off  latency=1  precision=Full  arith_type=Unsigned  n_bits=16  bin_pt=0  align_bp=on  dbl_ovrd=off  block_type=logical
      settings: block_version=12.1
  Register : xbsIndex_r4/Register  init=0  rst=off  en=on  dbl_ovrd=off  block_type=register
      settings: block_version=9.2.00
  Register{1..7} (7 alike) : xbsIndex_r4/Register  init=0  rst=on  en=off  dbl_ovrd=off  block_type=register
      settings: block_version=9.2.00
  Reinterpret : xbsIndex_r4/Reinterpret  force_arith_type=on  arith_type="Signed  (2's comp)"  force_bin_pt=on  bin_pt=16  block_type=reinterpret
      settings: infoedit="Changes signal type without altering the binary representation.   You can changed the signal between signed and unsigned, and relocate the binary point.<br><br>Hardware notes: In hardware this block costs nothing.<br><br>Example:  Suppose the input is 6 bits wide, signed, with 2 fractional bits, and the output is forced to unsigned with 0 fractional bits.  Then an input of -2.0 (1110.00 in binary 2's complement) becomes an output of 56 (111000 in binary)."  block_version=12.1
  Reset_Bit : xbsIndex_r4/Slice  nbits=1  boolean_output=on  mode=Lower Bit Location + Width  bit1=-17  base1=LSB of Input  bit0=2  base0=LSB of Input  dbl_ovrd=off  block_type=slice
      settings: block_version=12.1
  Terminator : Terminator
  Terminator1 : Terminator
  Write_Enable : xbsIndex_r4/Slice  nbits=1  boolean_output=on  mode=Lower Bit Location + Width  bit1=-17  base1=LSB of Input  bit0=1  base0=LSB of Input  dbl_ovrd=off  block_type=slice
      settings: block_version=12.1
  RX_I : Outport
  RX_Q : Outport  Port=2
  TX_I : Outport  Port=3
  TX_Q : Outport  Port=4
  Suppress_while_Tx : Outport  Port=5
  wires:
  Reset_Bit/1 -> 2 channel (IQ)  SHARED MPY MAC with Writable Coefficient Store/4(Reset)
  Write_Enable/1 -> Logical1/1
  Address_Slice/1 -> 2 channel (IQ)  SHARED MPY MAC with Writable Coefficient Store/6(Coef_RAM_Addr)
  WR_COEF_RAM/1 -> Logical/2, Register/2
  Register/1 -> Down Sample/1
  Down Sample/1 -> Data_Slice/1, Reset_Bit/1, Write_Enable/1, Address_Slice/1, Bank_Sel/1
  Data_Slice/1 -> Reinterpret/1
  Reinterpret/1 -> 2 channel (IQ)  SHARED MPY MAC with Writable Coefficient Store/5(Coef)
  Down Sample1/1 -> Register2/2, Logical1/2  "we"
  Logical/1 -> Register2/1
  Register2/1 -> Down Sample1/1, Logical/1
  Logical1/1 -> 2 channel (IQ)  SHARED MPY MAC with Writable Coefficient Store/8(we)
  Data_26/1 -> Register/1
  2 channel (IQ)  SHARED MPY MAC with Writable Coefficient Store/1(dout_1) -> Register1/1, Register6/1
  2 channel (IQ)  SHARED MPY MAC with Writable Coefficient Store/2(dout_2) -> Register3/1, Register7/1
  2 channel (IQ)  SHARED MPY MAC with Writable Coefficient Store/3(Addr_Out) -> Terminator1/1
  2 channel (IQ)  SHARED MPY MAC with Writable Coefficient Store/4(Coef_Out) -> Terminator/1
  Register1/1 -> TX_I/1
  Register3/1 -> TX_Q/1
  Tx_Rx_Delayed/1 -> Information_Filter_Transient_Suppressor/1(Tx_Rx_Delayed), 2 channel (IQ)  SHARED MPY MAC with Writable Coefficient Store/1(Tx_Rx_Delayed)
  Information_Filter_Transient_Suppressor/1(Supress_Tx_while_Rx) -> Register3/2, Register1/2
  Register4/1 -> 2 channel (IQ)  SHARED MPY MAC with Writable Coefficient Store/3(din2)
  Q_In/1 -> Register4/1
  Register5/1 -> 2 channel (IQ)  SHARED MPY MAC with Writable Coefficient Store/2(din1)
  I_In/1 -> Register5/1
  Information_Filter_Transient_Suppressor/3(Load Zeros) -> Register4/2, Register5/2
  Register7/1 -> RX_Q/1
  Register6/1 -> RX_I/1
  Information_Filter_Transient_Suppressor/2(Supress_Rx_while_Tx) -> Register6/2, Register7/2, Suppress_while_Tx/1
  Bank_Sel/1 -> 2 channel (IQ)  SHARED MPY MAC with Writable Coefficient Store/7(Bank_Sel)

== system Xcvr_SSB_AM_2p5/SSB / AM Mod_Demod WCS/Fixed Point HPF/LPF ==
  note: Was 1/128 but changed to
      | 1/256 to increase audio level.
  In1 : Inport
  Add : xbsIndex_r4/AddSub  mode=Addition  use_carryin=off  use_carryout=off  en=off  latency=0  precision=User Defined  arith_type=Unsigned  n_bits=32  bin_pt=26  quantization="Round  (unbiased: +/- Inf)"  overflow=Saturate  dbl_ovrd=off  use_behavioral_HDL=off  hw_selection=Fabric  pipelined=off  block_type=addsub
      settings: block_version=12.1
  CMult : xbsIndex_r4/CMult  const="1/256  % was 1/128"  gui_display_data_type=Fixed-point  const_n_bits=16  const_bin_pt=15  float_type=Single  exp_bits=8  fraction_bits=24  en=off  latency=1  precision=User Defined  arith_type=Unsigned  n_bits=16  bin_pt=15  quantization="Round  (unbiased: +/- Inf)"  overflow=Wrap  dbl_ovrd=off  use_behavioral_HDL=off  mem_type=Distributed RAM  pipeline=off  block_type=cmult
      settings: block_version=12.1
  CMult1 : xbsIndex_r4/CMult  const=1-1/128  gui_display_data_type=Fixed-point  const_n_bits=16  const_bin_pt=15  float_type=Single  exp_bits=8  fraction_bits=24  en=off  latency=0  precision=User Defined  arith_type=Unsigned  n_bits=32  bin_pt=26  quantization="Round  (unbiased: +/- Inf)"  overflow=Wrap  dbl_ovrd=off  use_behavioral_HDL=off  mem_type=Distributed RAM  pipeline=off  block_type=cmult
      settings: block_version=12.1
  Convert : xbsIndex_r4/Convert  gui_display_data_type=Fixed-point  arith_type="Signed  (2's comp)"  n_bits=16  bin_pt=15  float_type=Single  exp_bits=8  fraction_bits=24  quantization=Truncate  overflow=Wrap  en=off  latency=1  dbl_ovrd=off  pipeline=off  block_type=convert
      settings: block_version=12.1
  Delay1 : xbsIndex_r4/Delay  rst=off  infoeditControl=Selection of Reset will increase slice count due to use of real FFs and instead of SRLs  en=off  latency=1  dbl_ovrd=off  reg_retiming=off  block_type=delay
      settings: block_version=12.1
  Sub : xbsIndex_r4/AddSub  mode=Subtraction  use_carryin=off  use_carryout=off  en=off  latency=0  precision=User Defined  arith_type=Unsigned  n_bits=32  bin_pt=26  quantization=Truncate  overflow=Wrap  dbl_ovrd=off  use_behavioral_HDL=off  hw_selection=Fabric  pipelined=off  block_type=addsub
      settings: block_version=12.1
  Audio HPF : Outport
  Carrier Level LPF : Outport  Port=2
  wires:
  Sub/1 -> Convert/1
  CMult/1 -> Carrier Level LPF/1
  Add/1 -> Delay1/1, Sub/1
  Delay1/1 -> CMult1/1, CMult/1, Sub/2
  CMult1/1 -> Add/2
  In1/1 -> Add/1
  Convert/1 -> Audio HPF/1
